simulink library "SOMANETHandler"  (R2016b)
settings: Solver=VariableStepAuto  StartTime=0.0  StopTime=10.0  RelTol=1e-3
libraries: VariousLibrary x8, SOMANET x4
settings Model: Creator=Nathan  LastModifiedBy=MARCH

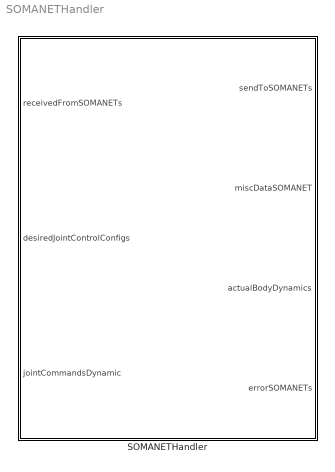
== system SOMANETHandler ==
  SOMANETHandler : Subsystem

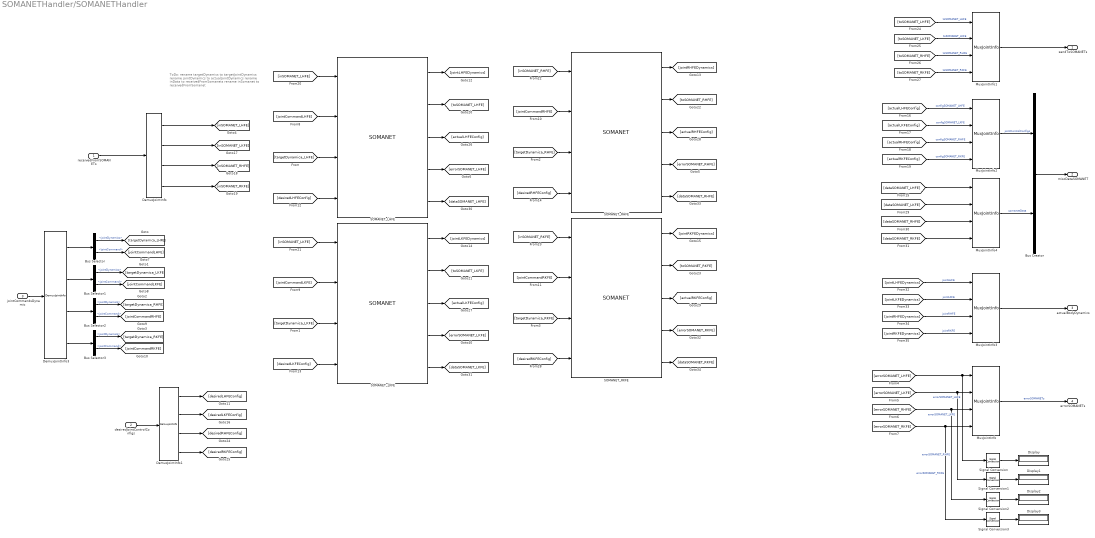
== system SOMANETHandler/SOMANETHandler ==
  note: ToDo: rename targetDynamics to targetJointDynamics
      | rename jointDynamics to actualJointDynamics
      | rename inData to receivedFromSomanets
      | rename inSomanet to receivedFromSomanet
  receivedFromSOMANETs : Inport  OutDataTypeStr=Bus: EtherCATReceivedFromSOMANET  PortDimensions=[1 4]  BusOutputAsStruct=on
  desiredJointControlConfigs : Inport  Port=2  OutDataTypeStr=Bus: JointControlConfig  PortDimensions=[1 4]
  jointCommandsDynamic : Inport  Port=3  OutDataTypeStr=Bus: JointDynamicCommand  PortDimensions=[1 4]
  Bus Creator : BusCreator  Inputs=2  OutDataTypeStr=Bus: MiscDataSOMANET  NonVirtualBus=on
  Bus Selector{,1..3} (4 alike) : BusSelector  OutputSignals=jointDynamics,jointCommand
  DemuxJointInfo : VariousLibrary/DemuxJointInfo
  DemuxJointInfo1 : VariousLibrary/DemuxJointInfo
  DemuxJointInfo3 : VariousLibrary/DemuxJointInfo
  Display{,1..3} (4 alike) : Display
  MuxJointInfo{,1..4} (5 alike) : VariousLibrary/MuxJointInfo
  SOMANET_LHFE : SOMANET/SOMANET
  SOMANET_LKFE : SOMANET/SOMANET
  SOMANET_RHFE : SOMANET/SOMANET
  SOMANET_RKFE : SOMANET/SOMANET
  Signal Conversion{,1..3} (4 alike) : SignalConversion  OverrideOpt=off
  sendToSOMANETs : Outport  OutDataTypeStr=Bus: EtherCATSendToSOMANET  PortDimensions=[1 4]  BusOutputAsStruct=on
  miscDataSOMANET : Outport  Port=2
  actualBodyDynamics : Outport  Port=3
  errorSOMANETs : Outport  Port=4  OutDataTypeStr=Enum: SomanetError  PortDimensions=[1 4]  BusOutputAsStruct=on
  wires:
  Signal Conversion3/1 -> Display3/1
  Signal Conversion2/1 -> Display2/1
  Signal Conversion1/1 -> Display1/1
  Signal Conversion/1 -> Display/1
  MuxJointInfo4/1 -> Bus Creator/2  "somanetData"
  MuxJointInfo2/1 -> Bus Creator/1  "jointControlConfigs"
  [dataSOMANET_RKFE] -> MuxJointInfo4/4
  [dataSOMANET_RHFE] -> MuxJointInfo4/3
  [dataSOMANET_LKFE] -> MuxJointInfo4/2
  [dataSOMANET_LHFE] -> MuxJointInfo4/1
  SOMANET_RKFE/5 -> [dataSOMANET_RKFE]
  SOMANET_RHFE/5 -> [dataSOMANET_RHFE]
  SOMANET_LKFE/5 -> [dataSOMANET_LKFE]
  SOMANET_LHFE/5 -> [dataSOMANET_LHFE]
  [errorSOMANET_LKFE] -> MuxJointInfo/2, Signal Conversion1/1  "errorSOMANET_LKFE"
  [errorSOMANET_RKFE] -> MuxJointInfo/4, Signal Conversion3/1  "errorSOMANET_RKFE"
  [errorSOMANET_RHFE] -> MuxJointInfo/3, Signal Conversion2/1  "errorSOMANET_RHFE"
  [errorSOMANET_LHFE] -> MuxJointInfo/1, Signal Conversion/1  "errorSOMANET_LHFE"
  MuxJointInfo/1 -> errorSOMANETs/1  "errorSOMANETs"
  [targetDynamica_RKFE] -> SOMANET_RKFE/3
  [targetDynamica_RHFE] -> SOMANET_RHFE/3
  [targetDynamica_LKFE] -> SOMANET_LKFE/3
  [toSOMANET_RHFE] -> MuxJointInfo1/3  "toSOMANET_RHFE"
  [toSOMANET_RKFE] -> MuxJointInfo1/4  "toSOMANET_RKFE"
  [toSOMANET_LKFE] -> MuxJointInfo1/2  "toSOMANET_LKFE"
  [inSOMANET_RKFE] -> SOMANET_RKFE/1
  [actualLKFEConfig] -> MuxJointInfo2/2  "configSOMANET_LKFE"
  [actualLHFEConfig] -> MuxJointInfo2/1  "configSOMANET_LHFE"
  [toSOMANET_LHFE] -> MuxJointInfo1/1  "toSOMANET_LHFE"
  MuxJointInfo1/1 -> sendToSOMANETs/1
  [inSOMANET_RHFE] -> SOMANET_RHFE/1
  [inSOMANET_LKFE] -> SOMANET_LKFE/1
  [inSOMANET_LHFE] -> SOMANET_LHFE/1
  [actualRKFEConfig] -> MuxJointInfo2/4  "configSOMANET_RKFE"
  [actualRHFEConfig] -> MuxJointInfo2/3  "configSOMANET_RHFE"
  Bus Creator/1 -> miscDataSOMANET/1
  SOMANET_RHFE/1 -> [jointRHFEDynamics]
  SOMANET_LKFE/1 -> [jointLKFEDynamics]
  SOMANET_RKFE/1 -> [jointRKFEDynamics]
  SOMANET_RHFE/2 -> [toSOMANET_RHFE]
  SOMANET_RHFE/3 -> [actualRHFEConfig]
  SOMANET_RHFE/4 -> [errorSOMANET_RHFE]
  SOMANET_RKFE/2 -> [toSOMANET_RKFE]
  SOMANET_RKFE/3 -> [actualRKFEConfig]
  SOMANET_RKFE/4 -> [errorSOMANET_RKFE]
  SOMANET_LKFE/2 -> [toSOMANET_LKFE]
  SOMANET_LKFE/3 -> [actualLKFEConfig]
  SOMANET_LKFE/4 -> [errorSOMANET_LKFE]
  [jointLHFEDynamics] -> MuxJointInfo3/1  "jointLHFE"
  [jointLKFEDynamics] -> MuxJointInfo3/2  "jointLKFE"
  [jointRHFEDynamics] -> MuxJointInfo3/3  "jointRHFE"
  [jointRKFEDynamics] -> MuxJointInfo3/4  "jointRKFE"
  MuxJointInfo3/1 -> actualBodyDynamics/1
  [jointCommandLHFE] -> SOMANET_LHFE/2
  [jointCommandLKFE] -> SOMANET_LKFE/2
  [jointCommandRHFE] -> SOMANET_RHFE/2
  [jointCommandRKFE] -> SOMANET_RKFE/2
  desiredJointControlConfigs/1 -> DemuxJointInfo1/1
  DemuxJointInfo1/4 -> [desiredRKFEConfig]
  DemuxJointInfo1/3 -> [desiredRHFEConfig]
  DemuxJointInfo1/2 -> [desiredLKFEConfig]
  DemuxJointInfo1/1 -> [desiredLHFEConfig]
  [desiredLKFEConfig] -> SOMANET_LKFE/4
  [desiredRHFEConfig] -> SOMANET_RHFE/4
  [desiredRKFEConfig] -> SOMANET_RKFE/4
  receivedFromSOMANETs/1 -> DemuxJointInfo/1
  DemuxJointInfo/4 -> [inSOMANET_RKFE]
  DemuxJointInfo/2 -> [inSOMANET_LKFE]
  DemuxJointInfo/3 -> [inSOMANET_RHFE]
  DemuxJointInfo/1 -> [inSOMANET_LHFE]
  [desiredLHFEConfig] -> SOMANET_LHFE/4
  [targetDynamica_LHFE] -> SOMANET_LHFE/3
  SOMANET_LHFE/1 -> [jointLHFEDynamics]
  SOMANET_LHFE/2 -> [toSOMANET_LHFE]
  SOMANET_LHFE/3 -> [actualLHFEConfig]
  SOMANET_LHFE/4 -> [errorSOMANET_LHFE]
  jointCommandsDynamic/1 -> DemuxJointInfo3/1
  DemuxJointInfo3/1 -> Bus Selector/1
  DemuxJointInfo3/2 -> Bus Selector1/1
  DemuxJointInfo3/3 -> Bus Selector2/1
  DemuxJointInfo3/4 -> Bus Selector3/1
  Bus Selector/2 -> [jointCommandLHFE]  "<jointCommand>"
  Bus Selector/1 -> [targetDynamica_LHFE]  "<jointDynamics>"
  Bus Selector1/2 -> [jointCommandLKFE]  "<jointCommand>"
  Bus Selector1/1 -> [targetDynamica_LKFE]  "<jointDynamics>"
  Bus Selector2/1 -> [targetDynamica_RHFE]  "<jointDynamics>"
  Bus Selector2/2 -> [jointCommandRHFE]  "<jointCommand>"
  Bus Selector3/2 -> [jointCommandRKFE]  "<jointCommand>"
  Bus Selector3/1 -> [targetDynamica_RKFE]  "<jointDynamics>"
